simulink subsystem "RT_SkewCalculation"  (R2025a)
settings: Solver=VariableStepAuto  StartTime=0.0  StopTime=2  RelTol=1e-3
settings Model: Creator=Admin  LastModifiedBy=Admin
settings DataIOCC: OutputSaveName=simout

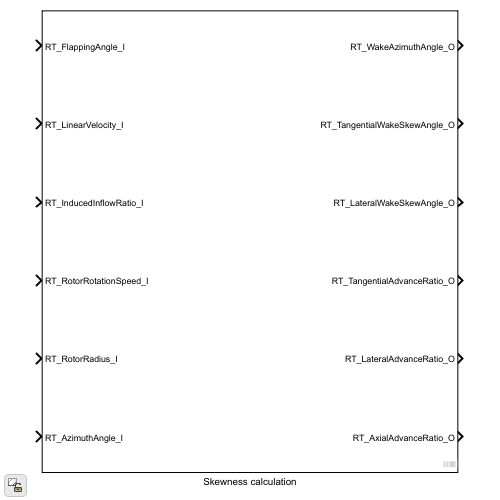
[thumbnail: Simulink's stored preview of the top-level diagram]
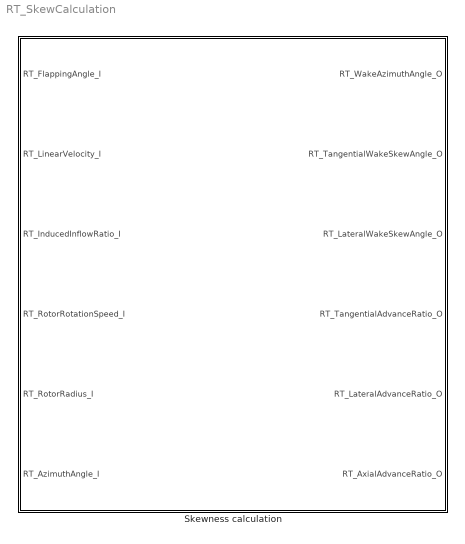
== system RT_SkewCalculation ==
  Skewness calculation : Subsystem

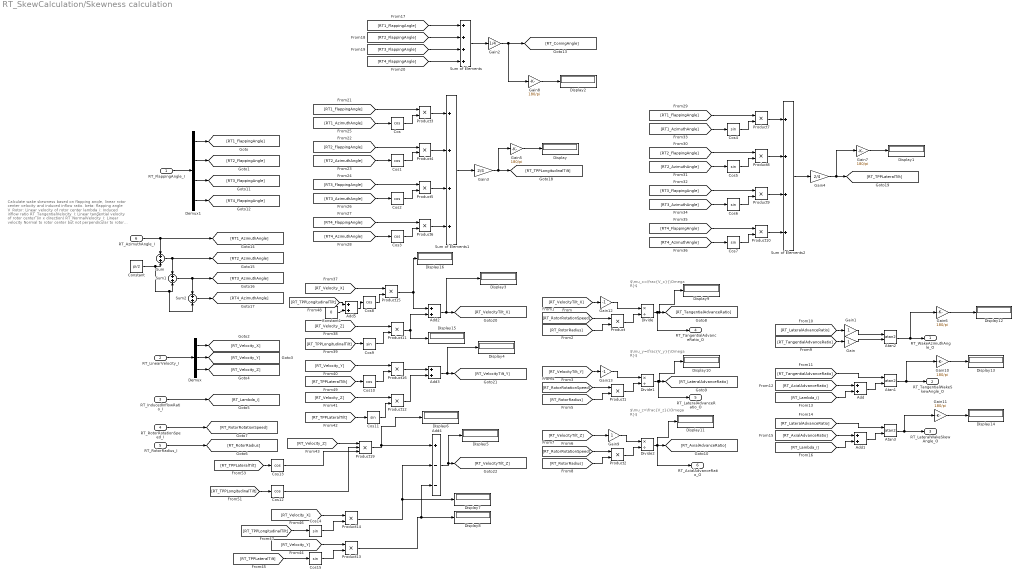
== system RT_SkewCalculation/Skewness calculation ==
  note: $\mu_x=\frac{V_x}{\Omega R}$
  note: Calculate wake skewness based on flapping angle, linear rotor center velocity and induced inflow ratio.
      |
      | beta: flapping angle
      | V_Rotor: Linear velocity of rotor center
      | lambda_i: Induced inflow ratio
      | RT_TangentialVelocity_I: Linear tangential velocity of rotor center (in x direction)
      | RT_NormalVelocity_I: Linear velocity Normal to rotor center but not perpendicular to rotor plane (y direction for MR and z direction for TR)
      |
      | chi: Wake skew angle
      | mu_x: advance ratio in longitudinal direction
      | mu_y: advance ratio in lateral direction
  note: $\mu_y=\frac{V_y}{\Omega R}$
  note: $\mu_z=\frac{V_z}{\Omega R}$
  RT_FlappingAngle_I : Inport
  RT_LinearVelocity_I : Inport  Port=2
  RT_InducedInflowRatio_I : Inport  Port=3
  RT_RotorRotationSpeed_I : Inport  Port=4
  RT_RotorRadius_I : Inport  Port=5
  RT_AzimuthAngle_I : Inport  Port=6
  Add{,1..3,5} (5 alike) : Sum
  Add4 : Sum  Inputs=+--
  Atan1 : Trigonometry  Operator=atan2
  Atan2 : Trigonometry  Operator=atan2
  Atan3 : Trigonometry  Operator=atan2
  Constant : Constant  Value=pi/2
  Constant1 : Constant  Value=0
  Cos{,1..3,8,10,12..13} (8 alike) : Trigonometry  Operator=cos
  Cos{4..7,9,11,14..15} (8 alike) : Trigonometry
  Demux : Demux  Outputs=3
  Demux1 : Demux
  Display{,1..16} (17 alike) : Display
  Divide : Product  Inputs=*/
  Divide1 : Product  Inputs=*/
  Divide2 : Product  Inputs=*/
  Gain : Gain
  Gain1 : Gain
  Gain{5..8,10..11} (6 alike) : Gain  Gain=180/pi
  Gain12 : Gain  Gain=-1
  Gain13 : Gain  Gain=-1
  Gain2 : Gain  Gain=1/4
  Gain3 : Gain  Gain=2/4
  Gain4 : Gain  Gain=2/4
  Gain9 : Gain
  Product{,1..16} (17 alike) : Product
  Product19 : Product  Inputs=3
  Sum : Sum
  Sum of Elements : Sum  Inputs=++++
  Sum of Elements1 : Sum  Inputs=++++
  Sum of Elements2 : Sum  Inputs=++++
  Sum1 : Sum
  Sum2 : Sum
  RT_WakeAzimuthAngle_O : Outport
  RT_TangentialWakeSkewAngle_O : Outport  Port=2
  RT_LateralWakeSkewAngle_O : Outport  Port=3
  RT_TangentialAdvanceRatio_O : Outport  Port=4
  RT_LateralAdvanceRatio_O : Outport  Port=5
  RT_AxialAdvanceRatio_O : Outport  Port=6
  wires:
  Gain13/1 -> Divide1/1
  Gain12/1 -> Divide/1
  Constant1/1 -> Add5/2
  [RT_TPPLongitudinalTilt] -> Add5/1
  Add5/1 -> Cos8/1
  Cos13/1 -> Product19/3
  Gain11/1 -> Display14/1
  Gain10/1 -> Display13/1
  Gain6/1 -> Display12/1
  Gain9/1 -> Divide2/1
  Cos15/1 -> Product13/2
  Cos14/1 -> Product14/2
  Product19/1 -> Add4/1, Display6/1
  [RT_Velocity_Z] -> Product19/1
  [RT_TPPLateralTilt] -> Cos13/1
  [RT_TPPLongitudinalTilt] -> Cos12/1
  Cos12/1 -> Product19/2
  Cos11/1 -> Product12/2
  Cos10/1 -> Product16/2
  [RT_TPPLateralTilt] -> Cos10/1
  [RT_Velocity_Y] -> Product16/1
  Product16/1 -> Add3/1
  Cos9/1 -> Product11/2
  [RT_TPPLongitudinalTilt] -> Cos9/1
  Cos8/1 -> Product15/2
  Product15/1 -> Add2/1, Display16/1
  [RT_Velocity_X] -> Product15/1
  Gain8/1 -> Display2/1
  Gain7/1 -> Display1/1
  Gain5/1 -> Display/1
  RT_RotorRadius_I/1 -> [RT_RotorRadius]
  Gain1/1 -> Atan2/1
  RT_RotorRotationSpeed_I/1 -> [RT_RotorRotationSpeed]
  RT_LinearVelocity_I/1 -> Demux/1
  Demux/1 -> [RT_Velocity_X]
  Demux/2 -> [RT_Velocity_Y]
  Demux/3 -> [RT_Velocity_Z]
  RT_InducedInflowRatio_I/1 -> [RT_Lambda_i]
  Demux1/1 -> [RT1_FlappingAngle]
  Demux1/2 -> [RT2_FlappingAngle]
  RT_FlappingAngle_I/1 -> Demux1/1
  [RT_RotorRotationSpeed] -> Product/1
  [RT_RotorRadius] -> Product/2
  Product/1 -> Divide/2
  [RT_VelocityTilt_X] -> Gain12/1
  Divide/1 -> RT_TangentialAdvanceRatio_O/1, [RT_TangentialAdvanceRatio], Display9/1
  [RT_VelocityTilt_Y] -> Gain13/1
  Product1/1 -> Divide1/2
  [RT_RotorRotationSpeed] -> Product1/1
  Divide1/1 -> RT_LateralAdvanceRatio_O/1, [RT_LateralAdvanceRatio], Display10/1
  [RT_RotorRadius] -> Product1/2
  [RT_RotorRadius] -> Product2/2
  [RT_RotorRotationSpeed] -> Product2/1
  Divide2/1 -> [RT_AxialAdvanceRatio], RT_AxialAdvanceRatio_O/1, Display11/1
  [RT_VelocityTilt_Z] -> Gain9/1
  Product2/1 -> Divide2/2
  [RT_TangentialAdvanceRatio] -> Gain/1
  [RT_LateralAdvanceRatio] -> Gain1/1
  Gain/1 -> Atan2/2
  Atan2/1 -> RT_WakeAzimuthAngle_O/1, Gain6/1
  [RT_AxialAdvanceRatio] -> Add/1
  Atan1/1 -> RT_TangentialWakeSkewAngle_O/1, Gain10/1
  [RT_TangentialAdvanceRatio] -> Atan1/1
  [RT_Lambda_i] -> Add/2
  Add/1 -> Atan1/2
  [RT_AxialAdvanceRatio] -> Add1/1
  [RT_Lambda_i] -> Add1/2
  Atan3/1 -> RT_LateralWakeSkewAngle_O/1, Gain11/1
  [RT_LateralAdvanceRatio] -> Atan3/1
  Add1/1 -> Atan3/2
  Demux1/3 -> [RT3_FlappingAngle]
  Demux1/4 -> [RT4_FlappingAngle]
  [RT1_FlappingAngle] -> Sum of Elements/1
  [RT2_FlappingAngle] -> Sum of Elements/2
  [RT3_FlappingAngle] -> Sum of Elements/3
  [RT4_FlappingAngle] -> Sum of Elements/4
  Sum of Elements/1 -> Gain2/1
  Gain2/1 -> [RT_ConingAngle], Gain8/1
  RT_AzimuthAngle_I/1 -> [RT1_AzimuthAngle], Sum/1
  Constant/1 -> Sum2/2, Sum1/2, Sum/2
  Sum/1 -> Sum1/1, [RT2_AzimuthAngle]
  Sum1/1 -> Sum2/1, [RT3_AzimuthAngle]
  Sum2/1 -> [RT4_AzimuthAngle]
  Sum of Elements1/1 -> Gain3/1
  Gain3/1 -> [RT_TPPLongitudinalTilt], Gain5/1
  [RT1_AzimuthAngle] -> Cos/1
  [RT1_FlappingAngle] -> Product3/1
  Product3/1 -> Sum of Elements1/1
  Cos/1 -> Product3/2
  [RT2_AzimuthAngle] -> Cos1/1
  Cos1/1 -> Product4/2
  Product4/1 -> Sum of Elements1/2
  [RT2_FlappingAngle] -> Product4/1
  [RT3_AzimuthAngle] -> Cos2/1
  Cos2/1 -> Product5/2
  Product5/1 -> Sum of Elements1/3
  [RT3_FlappingAngle] -> Product5/1
  [RT4_AzimuthAngle] -> Cos3/1
  Cos3/1 -> Product6/2
  Product6/1 -> Sum of Elements1/4
  [RT4_FlappingAngle] -> Product6/1
  Product7/1 -> Sum of Elements2/1
  Cos4/1 -> Product7/2
  Sum of Elements2/1 -> Gain4/1
  Gain4/1 -> [RT_TPPLateralTilt], Gain7/1
  [RT1_AzimuthAngle] -> Cos4/1
  Product10/1 -> Sum of Elements2/4
  Product9/1 -> Sum of Elements2/3
  [RT1_FlappingAngle] -> Product7/1
  Cos5/1 -> Product8/2
  [RT2_FlappingAngle] -> Product8/1
  Product8/1 -> Sum of Elements2/2
  [RT4_FlappingAngle] -> Product10/1
  [RT3_FlappingAngle] -> Product9/1
  [RT4_AzimuthAngle] -> Cos7/1
  [RT3_AzimuthAngle] -> Cos6/1
  [RT2_AzimuthAngle] -> Cos5/1
  Cos7/1 -> Product10/2
  Cos6/1 -> Product9/2
  [RT_Velocity_Z] -> Product11/1
  Product11/1 -> Add2/2, Display15/1
  Add2/1 -> [RT_VelocityTilt_X], Display3/1
  [RT_TPPLateralTilt] -> Cos11/1
  Add3/1 -> [RT_VelocityTilt_Y], Display4/1
  [RT_Velocity_Z] -> Product12/1
  Product12/1 -> Add3/2
  Add4/1 -> [RT_VelocityTilt_Z], Display5/1
  [RT_Velocity_Y] -> Product13/1
  [RT_TPPLateralTilt] -> Cos15/1
  Product13/1 -> Display8/1, Add4/3
  [RT_TPPLongitudinalTilt] -> Cos14/1
  [RT_Velocity_X] -> Product14/1
  Product14/1 -> Add4/2, Display7/1
